simulink model "differential_drive_robot_model"  (R2023a)
settings: Solver=FixedStepDiscrete  StartTime=0.0  StopTime=10.0  FixedStep=delta_time  RelTol=1e-3
model workspace (MAT data in the model file):
  TR = Simulink.Parameter
  TR.Value = 0.5
  TR.DataType = 'auto'
  TR.Complexity = 'real'
  TR.Dimensions = [1 1]
  delta_time = Simulink.Parameter
  delta_time.Value = 0.1
  delta_time.DataType = 'auto'
  delta_time.Complexity = 'real'
  delta_time.Dimensions = [1 1]
settings Model: Creator=tshintai  LastModifiedBy=fy153
settings OptimizationCC: DefaultParameterBehavior=Inlined  EnhancedBackFolding=on  PassReuseOutputArgsAs=Individual arguments  ZeroExternalMemoryAtStartup=off  ZeroInternalMemoryAtStartup=off  OptimizeBlockOrder=speed  DifferentSizesBufferReuse=on  OptimizationCustomize=off  EfficientTunableParamExpr=on
settings DebuggingCC: ParameterTunabilityLossMsg=error
settings SFSimCC: MATLABDynamicMemAlloc=off
settings RTWCC: Description=Embedded Coder  SystemTargetFile=ert.tlc  TemplateMakefile=ert_default_tmf  GenerateReport=on  LaunchReport=on  GenerateCodeMetricsReport=on
settings CodeAppCC: ForceParamTrailComments=on  IgnoreCustomStorageClasses=off  OperatorAnnotations=on  SimulinkDataObjDesc=on  SFDataObjDesc=on  InsertBlockDesc=on
settings ERTTargetCC: TargetLangStandard=C99 (ISO)  GenerateSampleERTMain=on  InlinedParameterPlacement=NonHierarchical  ERTCustomFileTemplate=example_file_process.tlc

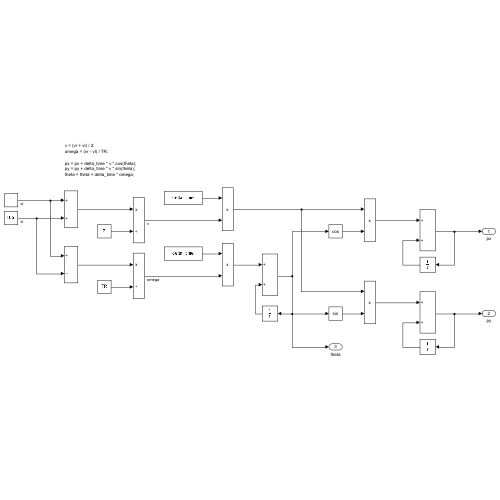
[thumbnail: Simulink's stored preview of the top-level diagram]
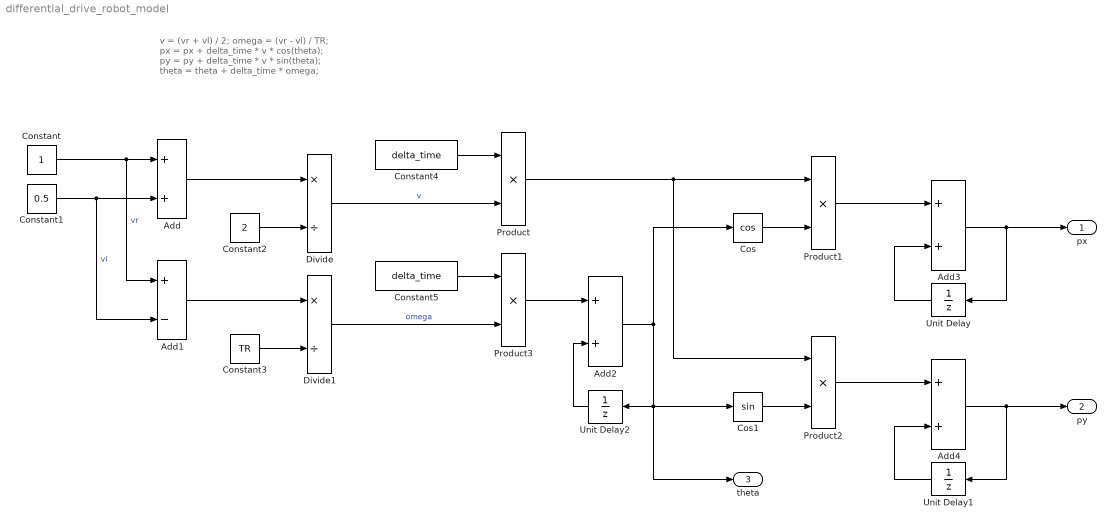
== system differential_drive_robot_model ==
  note: v = (vr + vl) / 2;
      | omega = (vr - vl) / TR;
      |
      | px = px + delta_time * v * cos(theta);
      | py = py + delta_time * v * sin(theta);
      | theta = theta + delta_time * omega;
  Add{,2..4} (4 alike) : Sum
  Add1 : Sum  Inputs=+-
  Constant : Constant
  Constant1 : Constant  Value=0.5
  Constant2 : Constant  Value=2
  Constant3 : Constant  Value=TR
  Constant4 : Constant  Value=delta_time
  Constant5 : Constant  Value=delta_time
  Cos : Trigonometry  Operator=cos
  Cos1 : Trigonometry
  Divide : Product  Inputs=*/
  Divide1 : Product  Inputs=*/
  Product{,1..3} (4 alike) : Product
  Unit Delay : UnitDelay  SampleTime=-1  HasFrameUpgradeWarning=on
  Unit Delay1 : UnitDelay  SampleTime=-1  HasFrameUpgradeWarning=on
  Unit Delay2 : UnitDelay  SampleTime=-1  HasFrameUpgradeWarning=on
  px : Outport
  py : Outport  Port=2
  theta : Outport  Port=3
  wires:
  Constant/1 -> Add1/1, Add/1  "vr"
  Constant1/1 -> Add/2, Add1/2  "vl"
  Add/1 -> Divide/1
  Constant2/1 -> Divide/2
  Constant3/1 -> Divide1/2
  Add1/1 -> Divide1/1
  Constant4/1 -> Product/1
  Divide/1 -> Product/2  "v"
  Cos/1 -> Product1/2
  Cos1/1 -> Product2/2
  Product/1 -> Product2/1, Product1/1
  Divide1/1 -> Product3/2  "omega"
  Constant5/1 -> Product3/1
  Product3/1 -> Add2/1
  Product1/1 -> Add3/1
  Unit Delay/1 -> Add3/2
  Add3/1 -> px/1, Unit Delay/1
  Add4/1 -> Unit Delay1/1, py/1
  Unit Delay1/1 -> Add4/2
  Product2/1 -> Add4/1
  Unit Delay2/1 -> Add2/2
  Add2/1 -> Cos/1, Cos1/1, Unit Delay2/1, theta/1
